simulink model "quadplane_control_dev"  (R2023a)
settings: Solver=FixedStepAuto  StartTime=0.0  StopTime=10.0  FixedStep=0.01  RelTol=1e-3
undefined symbols (not defined in the file or in its folder): Aircraft, DiscIntNeverNeededParam, framePeriod_s, frameRate_hz, InitCond
libraries: simulink x8, eeGeneralControl x6, slpidlib x3, fuzblock x1
(part 1 of 3)
settings Model: Creator=lagerprocessor  LastModifiedBy=redro
settings SolverCC: ZeroCrossControl=DisableAll
settings DataIOCC: SaveOutput=off  DSMLogging=off  SaveTime=off
settings DebuggingCC: ParameterPrecisionLossMsg=none
settings ModelReferenceCC: UseModelRefSolver=on
settings GRTTargetCC: CombineOutputUpdateFcns=off  MatFileLogging=off

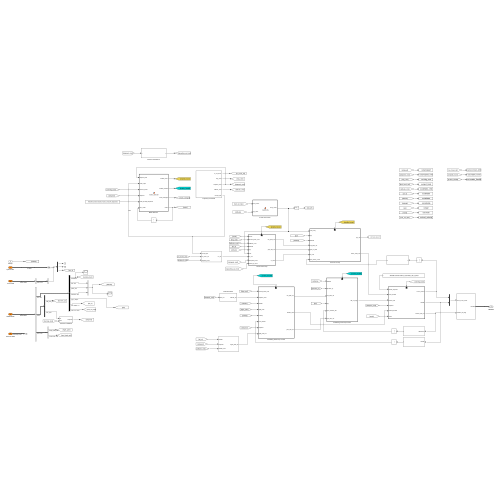
[thumbnail: Simulink's stored preview of the top-level diagram]
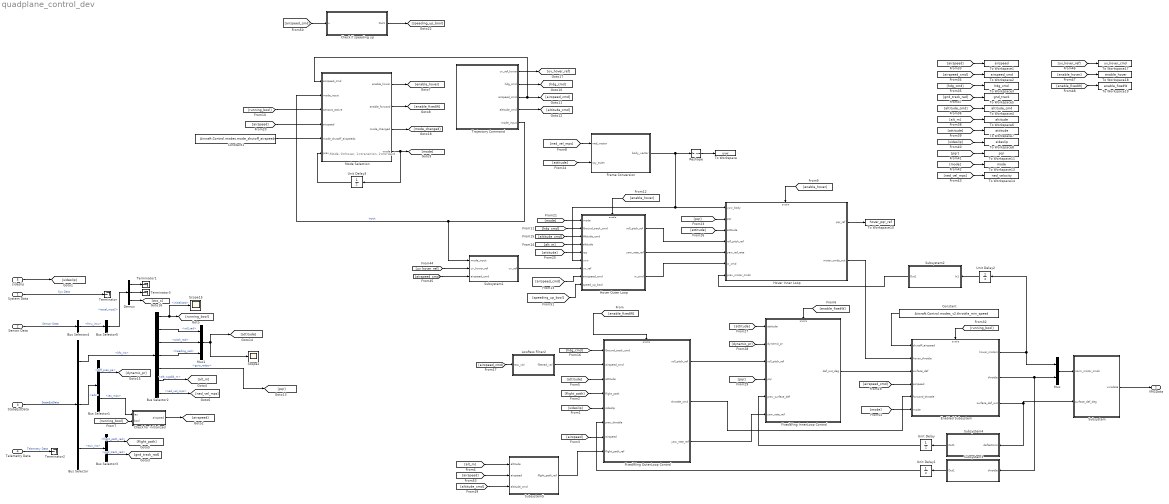
== system quadplane_control_dev ==
  note: Mode: 0=hover, 1=transition, 2=forward
  System Data : Inport  OutDataTypeStr=Bus: SysData  SampleTime=framePeriod_s  BusOutputAsStruct=on
  Sensor Data : Inport  Port=2  OutDataTypeStr=Bus: SensorData  SampleTime=framePeriod_s  BusOutputAsStruct=on
  StateEstData : Inport  Port=3  OutDataTypeStr=Bus: StateEstData  BusOutputAsStruct=on
  Telemetry Data : Inport  Port=4  OutDataTypeStr=Bus: TelemData  SampleTime=framePeriod_s  BusOutputAsStruct=on
  sideslip : Inport  Port=5  OutDataTypeStr=single
  Bus Selector : BusSelector  OutputSignals=bfs_ins,adc,aux_ins
  Bus Selector1 : BusSelector  OutputSignals=diff_pres_pa,ias_mps
  Bus Selector2 : BusSelector  OutputSignals=initialized,roll_rad,pitch_rad,heading_rad,gyro_radps,alt_wgs84_m,ned_vel_mps
  Bus Selector3 : BusSelector  OutputSignals=flight_path_rad,gnd_track_rad
  Bus Selector4 : BusSelector  OutputSignals=fmu_imu
  Bus Selector5 : BusSelector  OutputSignals=accel_mps2
  Check for initialized : Subsystem
  Check if speeding up : Subsystem
  Constant : Constant  Value=Aircraft.Control.modes_v2.throttle_min_speed
  Constant1 : Constant  Value=Aircraft.Control.modes.mode_shutoff_airspeeds
  Demux : Demux  Outputs=3
  Enabled Subsystem : Subsystem  TreatAsAtomicUnit=on
  FixedWing InnerLoop Control : Subsystem  TreatAsAtomicUnit=on
  FixedWing OuterLoop Control : Subsystem  TreatAsAtomicUnit=on
  Frame Conversion : MATLAB Function  TreatAsAtomicUnit=on
  Hover Inner Loop : Subsystem  TreatAsAtomicUnit=on
  Hover Outer Loop : Subsystem  TreatAsAtomicUnit=on
  LowPass Filter2 : Subsystem
      settings: PortSchema="{\"entries\":[{\"content\":{\"sides\":[{\"content\":{\"connectorIds\":[\"Out1\"]},\"type\":\"ConnectorPlacement.EquallySpacedRectSide\",\"uuid\":\"91cc3e13-2b14-472d-8884-d1975898cd34\"},{\"content\":{\"connectorIds\":[\"In1\"],\"side\":\"RIGHT\"},\"type\":\"ConnectorPlacement.EquallySpacedRectSide\",\"uuid\":\"ce6b3021-6e32-4737-8c8e-25014706d3dd\"},{\"content\":{\"side\":\"TOP\"},\"type\":\"ConnectorPlacement.EquallySpacedRectSide\",\"uuid\":\"ad734f0b-b067-43e6-a641-0e0955250a7f\"},{\"content\":{\"side\":\"BOTTOM\"},\"type\":\"ConnectorPlacement.EquallySpacedRectSide\",\"uuid\":\"618c62c8-d4e2-4678-9fe1-905e2f147d5d\"}]},\"type\":\"ConnectorPlacement.EquallySpacedConnector\",\"uuid\":\"c0097053-d36a-473a-84fb-0616f69f4bc5\"}],\"packageUris\":[\"http://schema.mathworks.com/mf0/Connector/R2020b\"],\"version\":\"1.0\"}"
  Mode Selection : MATLAB Function  TreatAsAtomicUnit=on
  Mux : Mux  Inputs=2
  Mux1 : Mux  Inputs=3
  Reshape : Reshape
  Scope15 : Scope
  Scope2 : Scope
  Subsystem : Subsystem
  Subsystem1 : Subsystem
  Subsystem2 : Subsystem
  Subsystem3 : Subsystem
  Subsystem4 : Subsystem
  Subsystem5 : Subsystem
  Terminator{,1..3} (4 alike) : Terminator
  To Workspace : ToWorkspace  VariableName=uvw  SampleTime=-1
      settings: Save2DSignal=2-D array (concatenate along first dimension)
  To Workspace1 : ToWorkspace  VariableName=airspeed  SaveFormat=Timeseries  SampleTime=-1
  To Workspace10 : ToWorkspace  VariableName=hover_pqr_ref  SaveFormat=Timeseries  SampleTime=-1
  To Workspace11 : ToWorkspace  VariableName=pqr  SaveFormat=Timeseries  SampleTime=-1
  To Workspace13 : ToWorkspace  VariableName=mode  SaveFormat=Timeseries  SampleTime=-1
  To Workspace14 : ToWorkspace  VariableName=ned_velocity  SaveFormat=Timeseries  SampleTime=-1
  To Workspace17 : ToWorkspace  VariableName=uv_hover_cmd  SaveFormat=Timeseries  SampleTime=-1
  To Workspace18 : ToWorkspace  VariableName=enable_hover  SaveFormat=Timeseries  SampleTime=-1
  To Workspace19 : ToWorkspace  VariableName=enable_fixedW  SaveFormat=Timeseries  SampleTime=-1
  To Workspace2 : ToWorkspace  VariableName=airspeed_cmd  SaveFormat=Timeseries  SampleTime=-1
  To Workspace3 : ToWorkspace  VariableName=hdg_cmd  SaveFormat=Timeseries  SampleTime=-1
  To Workspace4 : ToWorkspace  VariableName=altitude_cmd  SaveFormat=Timeseries  SampleTime=-1
  To Workspace5 : ToWorkspace  VariableName=gnd_track  SaveFormat=Timeseries  SampleTime=-1
  To Workspace6 : ToWorkspace  VariableName=altitude  SaveFormat=Timeseries  SampleTime=-1
  To Workspace7 : ToWorkspace  VariableName=attitude  SaveFormat=Timeseries  SampleTime=-1
  To Workspace8 : ToWorkspace  VariableName=sideslip  SaveFormat=Timeseries  SampleTime=-1
  Trajectory Command : Subsystem
  Unit Delay{,1..3} (4 alike) : UnitDelay  SampleTime=-1  HasFrameUpgradeWarning=on
  VMSData : Outport  OutDataTypeStr=Bus: VmsData
  wires:
  Telemetry Data/1 -> Terminator2/1  "Telemetry Data"
  StateEstData/1 -> Bus Selector/1  "StateEstData"
  Sensor Data/1 -> Bus Selector4/1  "Sensor Data"
  System Data/1 -> Terminator/1  "Sys Data"
  Subsystem/1(vmsdata) -> VMSData/1
  Bus Selector/2 -> Bus Selector1/1  "<adc>"
  Bus Selector/1 -> Bus Selector2/1  "<bfs_ins>"
  [enable_fixedW] -> FixedWing InnerLoop Control/Enable
  Bus Selector2/3 -> Mux1/2  "<pitch_rad>"
  Bus Selector2/4 -> Mux1/3  "<heading_rad>"
  Bus Selector/3 -> Bus Selector3/1  "<aux_ins>"
  Bus Selector4/1 -> Bus Selector5/1  "<fmu_imu>"
  Bus Selector5/1 -> Demux/1  "<accel_mps2>"
  Demux/1 -> Terminator1/1
  Demux/2 -> Terminator3/1
  sideslip/1 -> [sideslip]
  [sideslip] -> FixedWing OuterLoop Control/5(sideslip)
  Bus Selector2/1 -> Scope15/1, [running_bool]  "<initialized>"
  Bus Selector2/2 -> Mux1/1  "<roll_rad>"
  [hdg_cmd] -> FixedWing OuterLoop Control/1(Ground_track_cmd)
  Bus Selector3/2 -> [gnd_track_rad]  "<gnd_track_rad>"
  Bus Selector2/6 -> [alt_m]  "<alt_wgs84_m>"
  FixedWing OuterLoop Control/1(roll_pitch_ref) -> FixedWing InnerLoop Control/3(roll_pitch_ref)
  [airspeed_cmd] -> LowPass Filter2/1(raw_val)
  [flight_path] -> FixedWing OuterLoop Control/4(flight_path)
  [airspeed] -> FixedWing OuterLoop Control/7(airspeed)
  [attitude] -> FixedWing OuterLoop Control/3(attitude)
  [enable_fixedW] -> FixedWing OuterLoop Control/Enable
  Bus Selector2/7 -> [ned_vel_mps]  "<ned_vel_mps>"
  [ned_vel_mps] -> Frame Conversion/1(ned_vector)
  FixedWing InnerLoop Control/1(def_out_deg) -> Enabled Subsystem/3(surface_def)
  [enable_hover] -> Hover Inner Loop/Enable
  Hover Inner Loop/2(motor_cmds_out) -> Enabled Subsystem/2(hover_throttle)
  Hover Outer Loop/1(roll_pitch_ref) -> Hover Inner Loop/4(roll_pitch_ref)
  Hover Outer Loop/2(yaw_rate_ref) -> Hover Inner Loop/5(yaw_ref_rate)
  [enable_hover] -> Hover Outer Loop/Enable
  Hover Outer Loop/3(w_cmd) -> Hover Inner Loop/6(w_cmd)
  [hdg_cmd] -> Hover Outer Loop/2(Ground_track_cmd)
  [altitude_cmd] -> Hover Outer Loop/3(Altitude_cmd)
  [alt_m] -> Hover Outer Loop/4(altitude)
  Mode Selection/1(enable_hover) -> [enable_hover]
  Mode Selection/2(enable_forward) -> [enable_fixedW]
  [running_bool] -> Mode Selection/3(sensors_active)
  Trajectory Command/2(hdg_cmd) -> [hdg_cmd]
  Trajectory Command/4(altitude_cmd) -> [altitude_cmd]
  Trajectory Command/3(airspeed_cmd) -> Mode Selection/1(airspeed_cmd), [airspeed_cmd]
  [airspeed_cmd] -> Enabled Subsystem/4(airspeed)
  Mux/1 -> Subsystem/1(norm_motor_cmds)
  Enabled Subsystem/2(throttle) -> Subsystem3/1(throttle), Mux/2
  Unit Delay/1 -> FixedWing InnerLoop Control/5(prev_surface_def)
  Subsystem2/1(Out1) -> Hover Inner Loop/7(prev_motor_cmds)
  [airspeed] -> Mode Selection/4(airspeed)
  [mode] -> Hover Outer Loop/1(mode)
  Mode Selection/4(mode) -> Unit Delay3/1, [mode]
  Bus Selector2/5 -> [pqr]  "<gyro_radps>"
  Mux1/1 -> Scope2/1, [attitude]
  Bus Selector1/1 -> [dynamic_pr]  "<diff_pres_pa>"
  Bus Selector3/1 -> [flight_path]  "<flight_path_rad>"
  Demux/3 -> [acc_z]
  [attitude] -> Frame Conversion/2(rpy_euler)
  [attitude] -> Hover Outer Loop/5(rpy)
  [pqr] -> Hover Inner Loop/2(pqr)
  [attitude] -> Hover Inner Loop/3(attitude)
  [attitude] -> FixedWing InnerLoop Control/1(attitude)
  [dynamic_pr] -> FixedWing InnerLoop Control/2(dynamic_pr)
  [pqr] -> FixedWing InnerLoop Control/4(pqr)
  Bus Selector1/2 -> Check for initialized/1(ias)  "<ias_mps>"
  [running_bool] -> Enabled Subsystem/Enable
  Frame Conversion/1(body_vector) -> Reshape/1, Hover Inner Loop/1(uvw_body), Hover Outer Loop/6(uvw)
  [airspeed] -> To Workspace1/1
  [airspeed_cmd] -> To Workspace2/1
  [hdg_cmd] -> To Workspace3/1
  [altitude_cmd] -> To Workspace4/1
  [gnd_track_rad] -> To Workspace5/1
  [alt_m] -> To Workspace6/1
  [attitude] -> To Workspace7/1
  [sideslip] -> To Workspace8/1
  Hover Inner Loop/1(pqr_ref) -> To Workspace10/1
  [pqr] -> To Workspace11/1
  [mode] -> To Workspace13/1
  [ned_vel_mps] -> To Workspace14/1
  Trajectory Command/1(uv_ref_hover) -> [uv_hover_ref]
  Reshape/1 -> To Workspace/1
  Enabled Subsystem/1(hover_motors) -> Unit Delay2/1, Mux/1
  Enabled Subsystem/3(surface_def_out) -> Subsystem/2(surface_def_deg), Subsystem4/1(deflections)
  Subsystem1/1(uv_ref) -> Hover Outer Loop/7(uv_ref)
  [airspeed_cmd] -> Subsystem1/3(airspeed_cmd)
  [uv_hover_ref] -> Subsystem1/2(uv_hover_ref)
  [enable_hover] -> To Workspace18/1
  [enable_fixedW] -> To Workspace19/1
  [uv_hover_ref] -> To Workspace17/1
  FixedWing OuterLoop Control/3(yaw_rate_ref) -> FixedWing InnerLoop Control/6(yaw_rate_ref)
  Unit Delay2/1 -> Subsystem2/1(In1)
  Subsystem4/1(Out1) -> Unit Delay/1
  Unit Delay1/1 -> FixedWing OuterLoop Control/6(prev_throttle)
  Subsystem3/1(Out1) -> Unit Delay1/1
  Check for initialized/1(airspeed) -> [airspeed]
  [running_bool] -> Check for initialized/2(bool)
  Unit Delay3/1 -> Mode Selection/6(prev_mode)
  [mode] -> Enabled Subsystem/6(mode)
  Trajectory Command/5(mode_input) -> Subsystem1/1(mode_input), Mode Selection/2(mode_input)  "input"
  Mode Selection/3(mode_changed) -> [mode_changed]
  LowPass Filter2/1(filtered_val) -> FixedWing OuterLoop Control/2(airspeed_cmd)
  Constant/1 -> Enabled Subsystem/1(shutoff_airspeed)
  Constant1/1 -> Mode Selection/5(mode_shutoff_airspeeds)
  FixedWing OuterLoop Control/2(throttle_cmd) -> Enabled Subsystem/5(forward_throttle)
  [airspeed_cmd] -> Hover Outer Loop/8(airscpeed_cmd)
  [airspeed_cmd] -> Check if speeding up/1(u)
  Check if speeding up/1(Out1) -> [speeding_up_bool]
  [speeding_up_bool] -> Hover Outer Loop/9(speed_up_bool)
  [alt_m] -> Subsystem5/1(altitude)
  [altitude_cmd] -> Subsystem5/3(altitude_cmd)
  [airspeed] -> Subsystem5/2(airspeed)
  Subsystem5/1(flight_path_ref) -> FixedWing OuterLoop Control/8(flight_path_ref)

== system quadplane_control_dev/Check for initialized ==
  ias : Inport
  bool : Inport  Port=2
  Constant : Constant  Value=InitCond.body_vel_mps(1)  OutDataTypeStr=single
  Switch : Switch  Criteria=u2 > Threshold  SaturateOnIntegerOverflow=off  InputSameDT=off
  airspeed : Outport
  wires:
  ias/1 -> Switch/1
  bool/1 -> Switch/2  "bool"
  Constant/1 -> Switch/3
  Switch/1 -> airspeed/1

== system quadplane_control_dev/Check if speeding up ==
  u : Inport
  Constant2 : Constant  OutDataTypeStr=single
  Constant3 : Constant  Value=0  OutDataTypeStr=single
  Filtered Derivative (Discrete or Continuous) : eeGeneralControl/Filtered Derivative (Discrete or Continuous)  K=1  T=0.1  B=inf  A=-inf  minRatio=10  init_option=Inherited from block input  x0=0  Ts=-1
      settings: LibrarySourceBlock=|
      | ee_sl_lib/General Control/Filtered Derivative
      | (Discrete or Continuous)
  LowPass Filter : Subsystem
  Scope : Scope
  Switch : Switch  Criteria=u2 > Threshold  SaturateOnIntegerOverflow=off  InputSameDT=off
  Out1 : Outport
  wires:
  Filtered Derivative (Discrete or Continuous)/1 -> LowPass Filter/1(raw_val)
  Switch/1 -> Out1/1
  LowPass Filter/1(filtered_val) -> Scope/1, Switch/2
  Constant3/1 -> Switch/3
  Constant2/1 -> Switch/1
  u/1 -> Filtered Derivative (Discrete or Continuous)/1

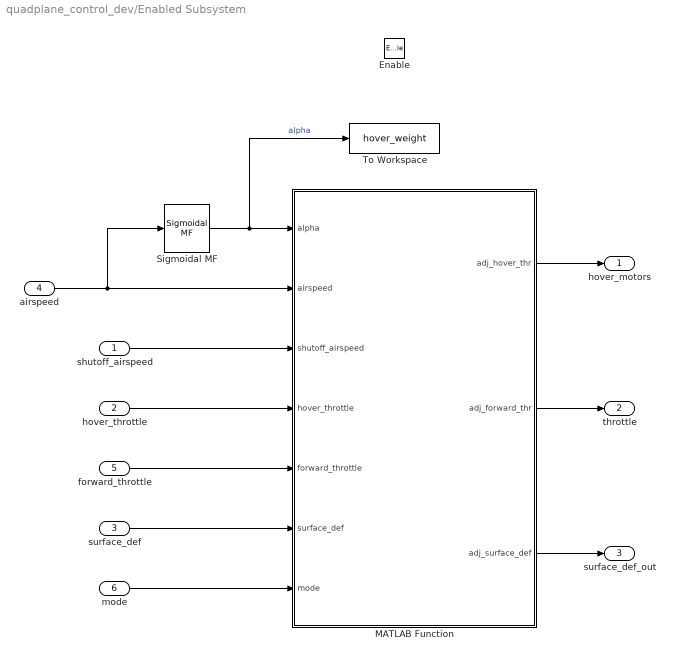
== system quadplane_control_dev/Enabled Subsystem ==
  shutoff_airspeed : Inport
  hover_throttle : Inport  Port=2
  surface_def : Inport  Port=3
  airspeed : Inport  Port=4
  forward_throttle : Inport  Port=5
  mode : Inport  Port=6
  Enable : EnablePort
  MATLAB Function : MATLAB Function  TreatAsAtomicUnit=on
  Sigmoidal MF : fuzblock/Membership  Functions/Sigmoidal MF  a=Aircraft.Control.modes_v2.transition_sigmoidal_a  c=Aircraft.Control.modes_v2.transition_sigmoidal_c
  To Workspace : ToWorkspace  VariableName=hover_weight  SaveFormat=Timeseries  SampleTime=-1
  hover_motors : Outport
  throttle : Outport  Port=2
  surface_def_out : Outport  Port=3
  wires:
  MATLAB Function/3(adj_surface_def) -> surface_def_out/1
  MATLAB Function/2(adj_forward_thr) -> throttle/1
  airspeed/1 -> Sigmoidal MF/1, MATLAB Function/2(airspeed)
  forward_throttle/1 -> MATLAB Function/5(forward_throttle)
  surface_def/1 -> MATLAB Function/6(surface_def)
  Sigmoidal MF/1 -> To Workspace/1, MATLAB Function/1(alpha)  "alpha"
  MATLAB Function/1(adj_hover_thr) -> hover_motors/1
  hover_throttle/1 -> MATLAB Function/4(hover_throttle)
  mode/1 -> MATLAB Function/7(mode)
  shutoff_airspeed/1 -> MATLAB Function/3(shutoff_airspeed)

== system quadplane_control_dev/FixedWing InnerLoop Control ==
  attitude : Inport
  dynamic_pr : Inport  Port=2
  roll_pitch_ref : Inport  Port=3
  pqr : Inport  Port=4
  prev_surface_def : Inport  Port=5
  yaw_rate_ref : Inport  Port=6
  Enable : EnablePort
  INDI Based Angular Rate Controller : Subsystem
  NDI based Attitude Controller : Subsystem
  To Workspace : ToWorkspace  VariableName=forward_pqr_cmd  SaveFormat=Timeseries  SampleTime=-1
  def_out_deg : Outport
  wires:
  dynamic_pr/1 -> INDI Based Angular Rate Controller/1(dynamic_pr)
  pqr/1 -> INDI Based Angular Rate Controller/3(pqr)
  attitude/1 -> NDI based Attitude Controller/1(attitude)
  NDI based Attitude Controller/1(pqr_ref) -> To Workspace/1, INDI Based Angular Rate Controller/2(pqr_ref)
  roll_pitch_ref/1 -> NDI based Attitude Controller/2(roll_pitch_ref)
  prev_surface_def/1 -> INDI Based Angular Rate Controller/4(prev_surface_def)
  INDI Based Angular Rate Controller/1(def_out_deg) -> def_out_deg/1
  yaw_rate_ref/1 -> NDI based Attitude Controller/3(yaw_rate_ref)

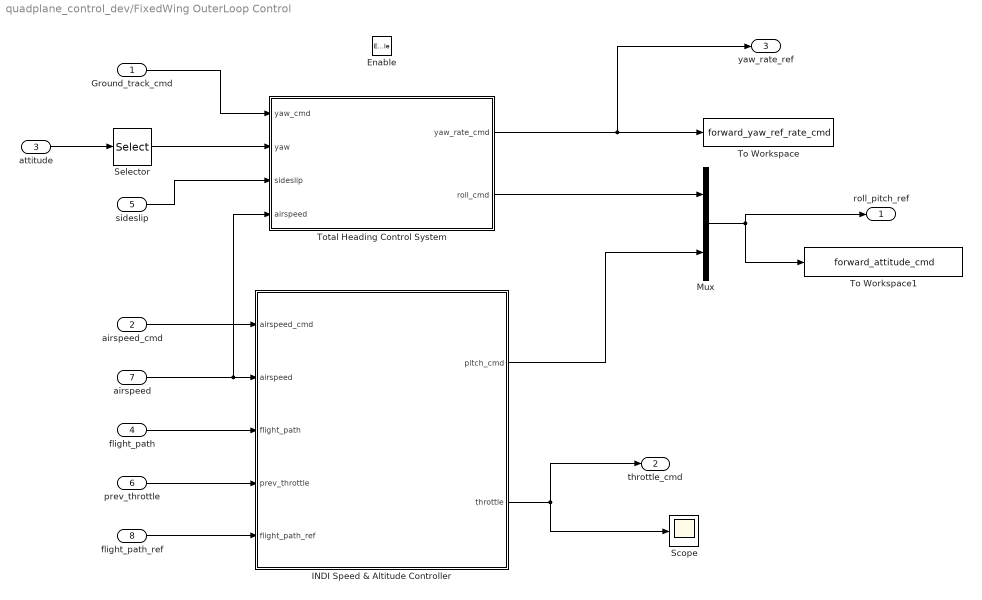
== system quadplane_control_dev/FixedWing OuterLoop Control ==
  Ground_track_cmd : Inport
  airspeed_cmd : Inport  Port=2
  attitude : Inport  Port=3
  flight_path : Inport  Port=4
  sideslip : Inport  Port=5
  prev_throttle : Inport  Port=6
  airspeed : Inport  Port=7
  flight_path_ref : Inport  Port=8
  Enable : EnablePort
  INDI Speed & Altitude Controller : Subsystem
  Mux : Mux  Inputs=2
  Scope : Scope
  Selector : Selector  InputPortWidth=3  IndexOptions=Index vector (dialog)  Indices=3  OutputSizes=1
  To Workspace : ToWorkspace  VariableName=forward_yaw_ref_rate_cmd  SaveFormat=Timeseries  SampleTime=-1
  To Workspace1 : ToWorkspace  VariableName=forward_attitude_cmd  SaveFormat=Timeseries  SampleTime=-1
  Total Heading Control System : Subsystem
  roll_pitch_ref : Outport
  throttle_cmd : Outport  Port=2
  yaw_rate_ref : Outport  Port=3
  wires:
  Ground_track_cmd/1 -> Total Heading Control System/1(yaw_cmd)
  INDI Speed & Altitude Controller/2(throttle) -> throttle_cmd/1, Scope/1
  flight_path/1 -> INDI Speed & Altitude Controller/3(flight_path)
  airspeed/1 -> Total Heading Control System/4(airspeed), INDI Speed & Altitude Controller/2(airspeed)
  Selector/1 -> Total Heading Control System/2(yaw)
  attitude/1 -> Selector/1
  sideslip/1 -> Total Heading Control System/3(sideslip)
  Mux/1 -> roll_pitch_ref/1, To Workspace1/1
  Total Heading Control System/2(roll_cmd) -> Mux/1
  Total Heading Control System/1(yaw_rate_cmd) -> yaw_rate_ref/1, To Workspace/1
  prev_throttle/1 -> INDI Speed & Altitude Controller/4(prev_throttle)
  airspeed_cmd/1 -> INDI Speed & Altitude Controller/1(airspeed_cmd)
  INDI Speed & Altitude Controller/1(pitch_cmd) -> Mux/2
  flight_path_ref/1 -> INDI Speed & Altitude Controller/5(flight_path_ref)

== system quadplane_control_dev/Hover Inner Loop ==
  uvw_body : Inport
  pqr : Inport  Port=2
  attitude : Inport  Port=3
  roll_pitch_ref : Inport  Port=4
  yaw_ref_rate : Inport  Port=5
  w_cmd : Inport  Port=6
  prev_motor_cmds : Inport  Port=7
  Enable : EnablePort
  Attitude Control : Subsystem
  INDI inner loop : Subsystem
  pqr_ref : Outport
  motor_cmds_out : Outport  Port=2
  wires:
  Attitude Control/1(pqr_ref1) -> pqr_ref/1, INDI inner loop/1(pqr_ref)
  uvw_body/1 -> INDI inner loop/2(uvw_body)
  pqr/1 -> INDI inner loop/4(pqr)
  INDI inner loop/1(motor_cmds_out) -> motor_cmds_out/1
  attitude/1 -> Attitude Control/3(roll_pitch_yaw)
  roll_pitch_ref/1 -> Attitude Control/2(roll_pitch_ref)
  prev_motor_cmds/1 -> INDI inner loop/5(prev_motor_cmds)
  w_cmd/1 -> INDI inner loop/3(w_ref)
  yaw_ref_rate/1 -> Attitude Control/1(yaw_rate_ref)

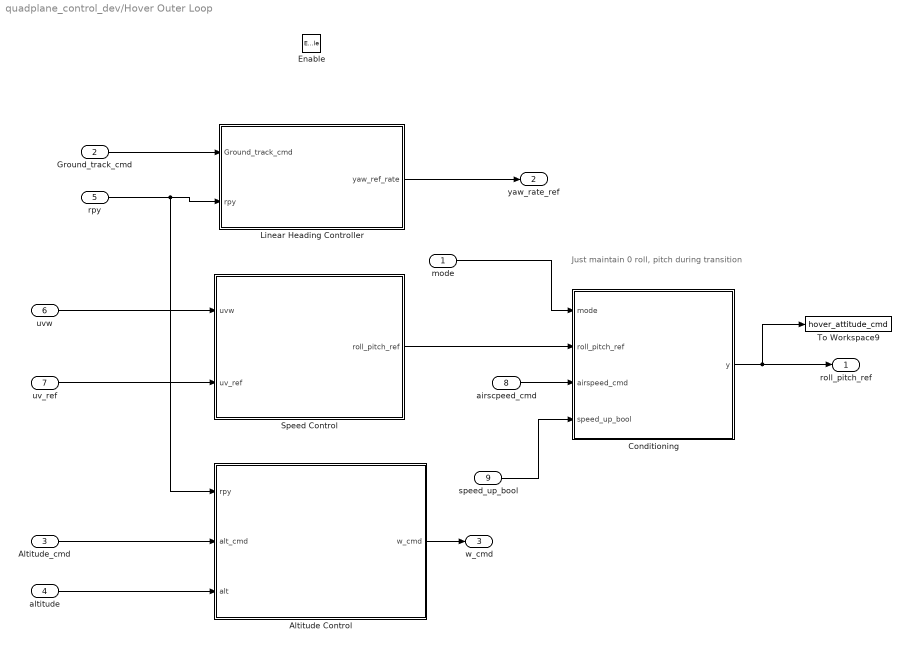
== system quadplane_control_dev/Hover Outer Loop ==
  note: Just maintain 0 roll, pitch during transition
  mode : Inport
  Ground_track_cmd : Inport  Port=2
  Altitude_cmd : Inport  Port=3
  altitude : Inport  Port=4
  rpy : Inport  Port=5
  uvw : Inport  Port=6
  uv_ref : Inport  Port=7
  airscpeed_cmd : Inport  Port=8
  speed_up_bool : Inport  Port=9
  Enable : EnablePort
  Altitude Control : Subsystem
  Conditioning : Subsystem
  Linear Heading Controller : Subsystem
  Speed Control : Subsystem
  To Workspace9 : ToWorkspace  VariableName=hover_attitude_cmd  SaveFormat=Timeseries  SampleTime=-1
  roll_pitch_ref : Outport
  yaw_rate_ref : Outport  Port=2
  w_cmd : Outport  Port=3
  wires:
  Altitude_cmd/1 -> Altitude Control/2(alt_cmd)
  altitude/1 -> Altitude Control/3(alt)
  rpy/1 -> Linear Heading Controller/2(rpy), Altitude Control/1(rpy)
  uvw/1 -> Speed Control/1(uvw)
  Speed Control/1(roll_pitch_ref) -> Conditioning/2(roll_pitch_ref)
  Altitude Control/1(w_cmd) -> w_cmd/1
  Conditioning/1(y) -> To Workspace9/1, roll_pitch_ref/1
  uv_ref/1 -> Speed Control/2(uv_ref)
  Linear Heading Controller/1(yaw_ref_rate) -> yaw_rate_ref/1
  Ground_track_cmd/1 -> Linear Heading Controller/1(Ground_track_cmd)
  mode/1 -> Conditioning/1(mode)
  airscpeed_cmd/1 -> Conditioning/3(airspeed_cmd)
  speed_up_bool/1 -> Conditioning/4(speed_up_bool)

== system quadplane_control_dev/LowPass Filter2 ==
  raw_val : Inport
  Constant : Constant  Value=Aircraft.Control.Forward_v2.airspeed_ref_LP_filter_CTOFF
  LP Filter on throttle outputs : Subsystem
      settings: PortSchema="{\"entries\":[{\"content\":{\"sides\":[{\"content\":{\"connectorIds\":[\"In1\"]},\"type\":\"ConnectorPlacement.EquallySpacedRectSide\",\"uuid\":\"20236834-aeb3-4c5b-bb2e-f84447e752b5\"},{\"content\":{\"connectorIds\":[\"Out1\"],\"side\":\"RIGHT\"},\"type\":\"ConnectorPlacement.EquallySpacedRectSide\",\"uuid\":\"d668f9a1-a3df-4207-8bf1-99fb838e59b2\"},{\"content\":{\"connectorIds\":[],\"side\":\"TOP\"},\"type\":\"ConnectorPlacement.EquallySpacedRectSide\",\"uuid\":\"66cceb06-f4bc-4278-b965-2427292e46df\"},{\"content\":{\"connectorIds\":[\"In2\"],\"side\":\"BOTTOM\"},\"type\":\"ConnectorPlacement.EquallySpacedRectSide\",\"uuid\":\"8fdaac6a-cb03-4bd4-87bb-7bafd10bc297\"}]},\"type\":\"ConnectorPlacement.EquallySpacedConnector\",\"uuid\":\"3dc29a9a-e794-478d-b7df-452e6c2d3f66\"}],\"packageUris\":[\"http://schema.mathworks.com/mf0/Connector/R2020b\"],\"version\":\"1.0\"}"
  To Workspace : ToWorkspace  VariableName=airspeed_ref  SaveFormat=Timeseries  SampleTime=-1
  filtered_val : Outport
  wires:
  raw_val/1 -> LP Filter on throttle outputs/1(raw_val)
  Constant/1 -> LP Filter on throttle outputs/2(freq_cut)
  LP Filter on throttle outputs/1(filtered_val) -> To Workspace/1, filtered_val/1

== system quadplane_control_dev/Subsystem ==
  note: norm_motor_cmds = [0,1]
  note: surface_def = [-30, 30]
  norm_motor_cmds : Inport
  surface_def_deg : Inport  Port=2
  Subsystem1 : Subsystem
  deflections_PWM_denormalize : Subsystem
  motor_PWM_denormalize : Subsystem
  vmsdata : Outport
  wires:
  motor_PWM_denormalize/1(raw_output) -> Subsystem1/1(Motor_Cmds)
  deflections_PWM_denormalize/1(raw_output) -> Subsystem1/2(Surface_def)
  Subsystem1/1(vmsdata) -> vmsdata/1
  norm_motor_cmds/1 -> motor_PWM_denormalize/1(normalized_input)
  surface_def_deg/1 -> deflections_PWM_denormalize/1(normalized_input)

== system quadplane_control_dev/Subsystem1 ==
  mode_input : Inport
  uv_hover_ref : Inport  Port=2
  airspeed_cmd : Inport  Port=3
  Constant : Constant  Value=0  OutDataTypeStr=single
  LowPass Filter1 : Subsystem
      settings: PortSchema="{\"entries\":[{\"content\":{\"sides\":[{\"content\":{\"connectorIds\":[\"Out1\"]},\"type\":\"ConnectorPlacement.EquallySpacedRectSide\",\"uuid\":\"91cc3e13-2b14-472d-8884-d1975898cd34\"},{\"content\":{\"connectorIds\":[\"In1\"],\"side\":\"RIGHT\"},\"type\":\"ConnectorPlacement.EquallySpacedRectSide\",\"uuid\":\"ce6b3021-6e32-4737-8c8e-25014706d3dd\"},{\"content\":{\"side\":\"TOP\"},\"type\":\"ConnectorPlacement.EquallySpacedRectSide\",\"uuid\":\"ad734f0b-b067-43e6-a641-0e0955250a7f\"},{\"content\":{\"side\":\"BOTTOM\"},\"type\":\"ConnectorPlacement.EquallySpacedRectSide\",\"uuid\":\"618c62c8-d4e2-4678-9fe1-905e2f147d5d\"}]},\"type\":\"ConnectorPlacement.EquallySpacedConnector\",\"uuid\":\"c0097053-d36a-473a-84fb-0616f69f4bc5\"}],\"packageUris\":[\"http://schema.mathworks.com/mf0/Connector/R2020b\"],\"version\":\"1.0\"}"
  Mux : Mux  Inputs=2
  Switch : Switch  Criteria=u2 > Threshold  SaturateOnIntegerOverflow=off  InputSameDT=off
  To Workspace : ToWorkspace  VariableName=uv_ref  SaveFormat=Timeseries  SampleTime=-1
  uv_ref : Outport
  wires:
  Switch/1 -> LowPass Filter1/1(raw_val)
  mode_input/1 -> Switch/2
  airspeed_cmd/1 -> Mux/1
  Constant/1 -> Mux/2
  Mux/1 -> Switch/1
  uv_hover_ref/1 -> Switch/3
  LowPass Filter1/1(filtered_val) -> To Workspace/1, uv_ref/1

== system quadplane_control_dev/Subsystem2 ==
  In1 : Inport
  Cast To Double : DataTypeConversion  OutDataTypeStr=double  SaturateOnIntegerOverflow=off  RndMeth=Floor
  Cast To Single : DataTypeConversion  OutDataTypeStr=single  SaturateOnIntegerOverflow=off  RndMeth=Floor
  Demux1 : Demux
  Mux2 : Mux
  Transfer Fcn{,1..3} (4 alike) : TransferFcn  Denominator=[1/Aircraft.Motor.bandwidth 1]
  Out1 : Outport
  wires:
  Transfer Fcn/1 -> Mux2/1
  Mux2/1 -> Cast To Single/1
  Transfer Fcn3/1 -> Mux2/4
  Demux1/2 -> Transfer Fcn1/1
  Demux1/3 -> Transfer Fcn2/1
  Demux1/4 -> Transfer Fcn3/1
  Transfer Fcn2/1 -> Mux2/3
  Transfer Fcn1/1 -> Mux2/2
  Demux1/1 -> Transfer Fcn/1
  In1/1 -> Cast To Double/1
  Cast To Double/1 -> Demux1/1
  Cast To Single/1 -> Out1/1

== system quadplane_control_dev/Subsystem3 ==
  throttle : Inport
  Cast To Double : DataTypeConversion  OutDataTypeStr=double  SaturateOnIntegerOverflow=off  RndMeth=Floor
  Cast To Single : DataTypeConversion  OutDataTypeStr=single  SaturateOnIntegerOverflow=off  RndMeth=Floor
  Transfer Fcn2 : TransferFcn  Denominator=[1/Aircraft.Motor.bandwidth 1]
  Out1 : Outport
  wires:
  throttle/1 -> Cast To Double/1
  Cast To Single/1 -> Out1/1
  Transfer Fcn2/1 -> Cast To Single/1
  Cast To Double/1 -> Transfer Fcn2/1

== system quadplane_control_dev/Subsystem4 ==
  deflections : Inport
  Cast To Double : DataTypeConversion  OutDataTypeStr=double  SaturateOnIntegerOverflow=off  RndMeth=Floor
  Cast To Single : DataTypeConversion  OutDataTypeStr=single  SaturateOnIntegerOverflow=off  RndMeth=Floor
  Demux : Demux  Outputs=3
  Mux : Mux  Inputs=3
  Transfer Fcn : TransferFcn  Denominator=[Aircraft.Surf.time_constant 1]
  Transfer Fcn1 : TransferFcn  Denominator=[Aircraft.Surf.time_constant 1]
  Transfer Fcn2 : TransferFcn  Denominator=[Aircraft.Surf.time_constant 1]
  Out1 : Outport
  wires:
  deflections/1 -> Cast To Double/1
  Cast To Single/1 -> Out1/1
  Transfer Fcn2/1 -> Mux/3
  Mux/1 -> Cast To Single/1
  Demux/2 -> Transfer Fcn1/1
  Demux/1 -> Transfer Fcn/1
  Transfer Fcn/1 -> Mux/1
  Demux/3 -> Transfer Fcn2/1
  Transfer Fcn1/1 -> Mux/2
  Cast To Double/1 -> Demux/1

== system quadplane_control_dev/Subsystem5 ==
  note: Converting from Alt_cmd to Flight_path_cmd
  altitude : Inport
  airspeed : Inport  Port=2
  altitude_cmd : Inport  Port=3
  Asin : Trigonometry  Operator=asin
  Divide : Product  Inputs=/*
  Gain : Gain  Gain=Aircraft.Control.Forward_v2.altitude_P
  LowPass Filter1 : Subsystem
      settings: PortSchema="{\"entries\":[{\"content\":{\"sides\":[{\"content\":{\"connectorIds\":[\"Out1\"]},\"type\":\"ConnectorPlacement.EquallySpacedRectSide\",\"uuid\":\"91cc3e13-2b14-472d-8884-d1975898cd34\"},{\"content\":{\"connectorIds\":[\"In1\"],\"side\":\"RIGHT\"},\"type\":\"ConnectorPlacement.EquallySpacedRectSide\",\"uuid\":\"ce6b3021-6e32-4737-8c8e-25014706d3dd\"},{\"content\":{\"side\":\"TOP\"},\"type\":\"ConnectorPlacement.EquallySpacedRectSide\",\"uuid\":\"ad734f0b-b067-43e6-a641-0e0955250a7f\"},{\"content\":{\"side\":\"BOTTOM\"},\"type\":\"ConnectorPlacement.EquallySpacedRectSide\",\"uuid\":\"618c62c8-d4e2-4678-9fe1-905e2f147d5d\"}]},\"type\":\"ConnectorPlacement.EquallySpacedConnector\",\"uuid\":\"c0097053-d36a-473a-84fb-0616f69f4bc5\"}],\"packageUris\":[\"http://schema.mathworks.com/mf0/Connector/R2020b\"],\"version\":\"1.0\"}"
  Saturation1 : Saturate  UpperLimit=4  LowerLimit=-4
  Sum : Sum  Inputs=|+-
  To Workspace : ToWorkspace  VariableName=flight_path_ref  SaveFormat=Timeseries  SampleTime=-1
  flight_path_ref : Outport
  wires:
  Saturation1/1 -> Divide/2  "h_dot_cmd"
  Sum/1 -> Gain/1  "alt_err"
  Asin/1 -> LowPass Filter1/1(raw_val)  "flight_path_cmd"
  altitude_cmd/1 -> Sum/1
  airspeed/1 -> Divide/1
  Gain/1 -> Saturation1/1  "alt_err"
  Divide/1 -> Asin/1
  altitude/1 -> Sum/2
  LowPass Filter1/1(filtered_val) -> To Workspace/1, flight_path_ref/1

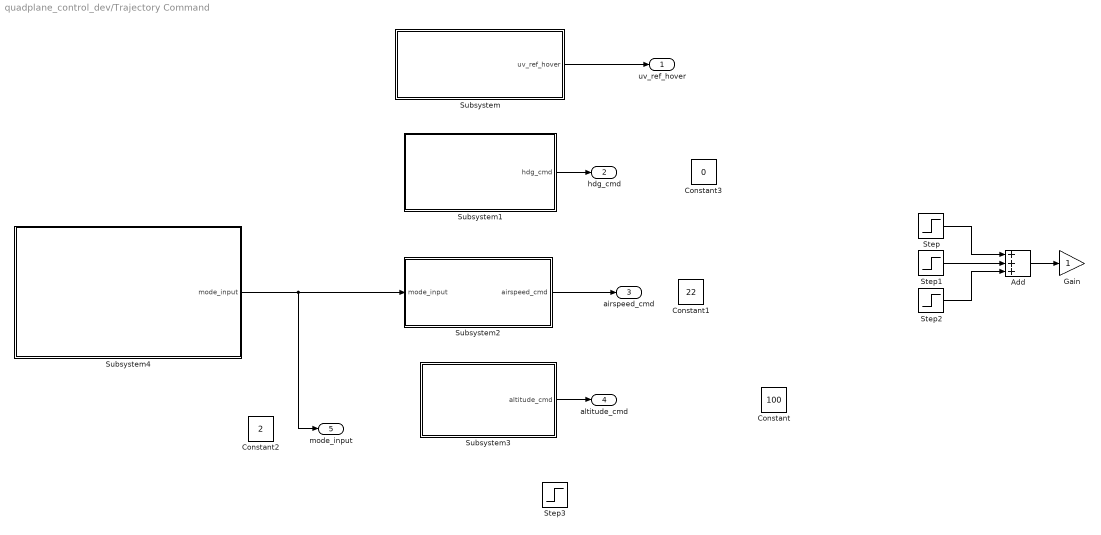
== system quadplane_control_dev/Trajectory Command ==
  Add : Sum  Inputs=+++
  Constant : Constant  Value=100  OutDataTypeStr=single
  Constant1 : Constant  Value=22  OutDataTypeStr=single
  Constant2 : Constant  Value=2  OutDataTypeStr=single
  Constant3 : Constant  Value=0  OutDataTypeStr=single
  Gain : Gain
  Step : Step  Time=6  OutDataTypeStr=single  SampleTime=0
  Step1 : Step  Time=12  Before=1  After=-1  OutDataTypeStr=single  SampleTime=0
  Step2 : Step  Time=18  Before=-1  After=0  OutDataTypeStr=single  SampleTime=0
  Step3 : Step  Time=3  Before=100  After=90  OutDataTypeStr=single  SampleTime=0
  Subsystem : Subsystem
  Subsystem1 : Subsystem
  Subsystem2 : Subsystem
  Subsystem3 : Subsystem
  Subsystem4 : Subsystem
  uv_ref_hover : Outport
  hdg_cmd : Outport  Port=2
  airspeed_cmd : Outport  Port=3
  altitude_cmd : Outport  Port=4
  mode_input : Outport  Port=5
  wires:
  Subsystem/1(uv_ref_hover) -> uv_ref_hover/1
  Subsystem3/1(altitude_cmd) -> altitude_cmd/1
  Subsystem4/1(mode_input) -> Subsystem2/1(mode_input), mode_input/1
  Subsystem2/1(airspeed_cmd) -> airspeed_cmd/1
  Subsystem1/1(hdg_cmd) -> hdg_cmd/1
  Step2/1 -> Add/3
  Step1/1 -> Add/2
  Step/1 -> Add/1
  Add/1 -> Gain/1

== system quadplane_control_dev/Check if speeding up/LowPass Filter ==
  raw_val : Inport
  Constant : Constant  Value=0.5  OutDataTypeStr=single
  LP Filter on Accel : Subsystem
      settings: PortSchema="{\"entries\":[{\"content\":{\"sides\":[{\"content\":{\"connectorIds\":[\"In1\"]},\"type\":\"ConnectorPlacement.EquallySpacedRectSide\",\"uuid\":\"20236834-aeb3-4c5b-bb2e-f84447e752b5\"},{\"content\":{\"connectorIds\":[\"Out1\"],\"side\":\"RIGHT\"},\"type\":\"ConnectorPlacement.EquallySpacedRectSide\",\"uuid\":\"d668f9a1-a3df-4207-8bf1-99fb838e59b2\"},{\"content\":{\"connectorIds\":[],\"side\":\"TOP\"},\"type\":\"ConnectorPlacement.EquallySpacedRectSide\",\"uuid\":\"66cceb06-f4bc-4278-b965-2427292e46df\"},{\"content\":{\"connectorIds\":[\"In2\"],\"side\":\"BOTTOM\"},\"type\":\"ConnectorPlacement.EquallySpacedRectSide\",\"uuid\":\"8fdaac6a-cb03-4bd4-87bb-7bafd10bc297\"}]},\"type\":\"ConnectorPlacement.EquallySpacedConnector\",\"uuid\":\"3dc29a9a-e794-478d-b7df-452e6c2d3f66\"}],\"packageUris\":[\"http://schema.mathworks.com/mf0/Connector/R2020b\"],\"version\":\"1.0\"}"
  filtered_val : Outport
  wires:
  raw_val/1 -> LP Filter on Accel/1(raw_val)
  Constant/1 -> LP Filter on Accel/2(freq_cut)
  LP Filter on Accel/1(filtered_val) -> filtered_val/1

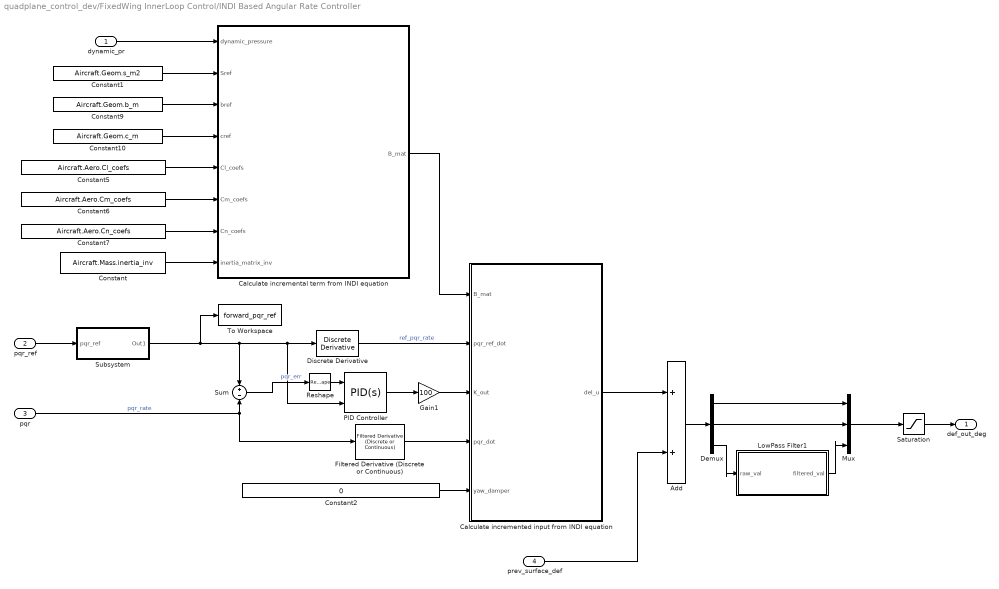
== system quadplane_control_dev/FixedWing InnerLoop Control/INDI Based Angular Rate Controller ==
  dynamic_pr : Inport
  pqr_ref : Inport  Port=2
  pqr : Inport  Port=3
  prev_surface_def : Inport  Port=4
  Add : Sum  OutDataTypeStr=single
  Calculate incremental term from INDI equation : MATLAB Function  TreatAsAtomicUnit=on
  Calculate incremented input from INDI equation : MATLAB Function  TreatAsAtomicUnit=on
  Constant : Constant  Value=Aircraft.Mass.inertia_inv  OutDataTypeStr=single
  Constant1 : Constant  Value=Aircraft.Geom.s_m2  OutDataTypeStr=single
  Constant10 : Constant  Value=Aircraft.Geom.c_m  OutDataTypeStr=single
  Constant2 : Constant  Value=0  OutDataTypeStr=single
  Constant5 : Constant  Value=Aircraft.Aero.Cl_coefs  OutDataTypeStr=single
  Constant6 : Constant  Value=Aircraft.Aero.Cm_coefs  OutDataTypeStr=single
  Constant7 : Constant  Value=Aircraft.Aero.Cn_coefs  OutDataTypeStr=single
  Constant9 : Constant  Value=Aircraft.Geom.b_m  OutDataTypeStr=single
  Demux : Demux  Outputs=3
  Discrete Derivative : simulink/Discrete/Discrete Derivative  gainval=1.0  ICPrevScaledInput=0.0  OutMin=[]  OutMax=[]  OutDataTypeStr=single  OutputDataTypeScalingMode=single  OutDataType=fixdt(1, 16)  OutScaling=2^-10  DoSatur=off
  Filtered Derivative (Discrete or Continuous) : eeGeneralControl/Filtered Derivative (Discrete or Continuous)  K=1  T=0.01  B=inf  A=-inf  minRatio=10  init_option=Inherited from block input  x0=0  Ts=-1
      settings: LibrarySourceBlock=|
      | ee_sl_lib/General Control/Filtered Derivative
      | (Discrete or Continuous)
  Gain1 : Gain  Gain=100
  LowPass Filter1 : Subsystem
      settings: PortSchema="{\"entries\":[{\"content\":{\"sides\":[{\"content\":{\"connectorIds\":[\"Out1\"]},\"type\":\"ConnectorPlacement.EquallySpacedRectSide\",\"uuid\":\"91cc3e13-2b14-472d-8884-d1975898cd34\"},{\"content\":{\"connectorIds\":[\"In1\"],\"side\":\"RIGHT\"},\"type\":\"ConnectorPlacement.EquallySpacedRectSide\",\"uuid\":\"ce6b3021-6e32-4737-8c8e-25014706d3dd\"},{\"content\":{\"side\":\"TOP\"},\"type\":\"ConnectorPlacement.EquallySpacedRectSide\",\"uuid\":\"ad734f0b-b067-43e6-a641-0e0955250a7f\"},{\"content\":{\"side\":\"BOTTOM\"},\"type\":\"ConnectorPlacement.EquallySpacedRectSide\",\"uuid\":\"618c62c8-d4e2-4678-9fe1-905e2f147d5d\"}]},\"type\":\"ConnectorPlacement.EquallySpacedConnector\",\"uuid\":\"c0097053-d36a-473a-84fb-0616f69f4bc5\"}],\"packageUris\":[\"http://schema.mathworks.com/mf0/Connector/R2020b\"],\"version\":\"1.0\"}"
  Mux : Mux  Inputs=3
  PID Controller : slpidlib/PID Controller  Controller=PID  Form=Parallel  TimeDomain=Continuous-time  UseExternalTs=off  SampleTime=-1  IntegratorMethod=Forward Euler  FilterMethod=Forward Euler  ControllerParametersSource=internal  P=[6, 6, 3]  I=[20, 20, 5]  UseKiTs=off  D=[0.5, 0.5, 0.75]  N=100  UseFilter=on  TunerSelectOption=Transfer Function Based (PID Tuner App)  InitialConditionSource=internal  InitialConditionForIntegrator=0  InitialConditionForFilter=0  DifferentiatorICPrevScaledInput=0  ExternalReset=none  TrackingMode=on  Kt=1  LimitOutput=off  SatLimitsSource=internal  UpperSaturationLimit=inf  LowerSaturationLimit=-inf  LinearizeAsGain=on  AntiWindupMode=none  Kb=1  LimitIntegrator=off  UpperIntegratorSaturationLimit=inf  LowerIntegratorSaturationLimit=-inf  POutMin=[]  POutMax=[]  IOutMin=[]  IOutMax=[]  DOutMin=[]  DOutMax=[]  NOutMin=[]  NOutMax=[]  SumOutMin=[]  SumOutMax=[]  SaturationOutMin=[]  SaturationOutMax=[]  PParamMin=[]  PParamMax=[]  IParamMin=[]  IParamMax=[]  DParamMin=[]  DParamMax=[]  NParamMin=[]  NParamMax=[]  KbParamMin=[]  KbParamMax=[]  KtParamMin=[]  KtParamMax=[]  KbOutMin=[]  KbOutMax=[]  KtOutMin=[]  KtOutMax=[]  IntegratorOutMin=[]  IntegratorOutMax=[]  FilterOutMin=[]  FilterOutMax=[]  SumI1OutMin=[]  SumI1OutMax=[]  SumI2OutMin=[]  SumI2OutMax=[]  SumI3OutMin=[]  SumI3OutMax=[]  SumI4OutMin=[]  SumI4OutMax=[]  SumDOutMin=[]  SumDOutMax=[]  DifferentiatorOutMin=[]  DifferentiatorOutMax=[]  FilterDiffOutCoefMin=[]  FilterDiffOutCoefMax=[]  ReciprocalOutMin=[]  ReciprocalOutMax=[]  SumDenOutMin=[]  SumDenOutMax=[]  SumNumOutMin=[]  SumNumOutMax=[]  DivideOutMin=[]  DivideOutMax=[]  UdiffTsProdOutMin=[]  UdiffTsProdOutMax=[]  NTsProdOutMin=[]  NTsProdOutMax=[]  UintegralTsProdOutMin=[]  UintegralTsProdOutMax=[]  UngainTsProdOutMin=[]  UngainTsProdOutMax=[]  ClampingZeroOutDataTypeStr=Inherit: Inherit via back propagation  ClampingZeroOutMin=[]  ClampingZeroOutMax=[]  FilterDenConstantOutDataTypeStr=Inherit: Inherit via back propagation  FilterDenConstantOutMin=[]  FilterDenConstantOutMax=[]  PCopyOutDataTypeStr=Inherit: Inherit via back propagation  PCopyOutMin=[]  PCopyOutMax=[]  NCopyOutDataTypeStr=Inherit: Inherit via back propagation  NCopyOutMin=[]  NCopyOutMax=[]  IntegratorContinuousStateAttributes=''  IntegratorStateMustResolveToSignalObject=off  IntegratorRTWStateStorageClass=Auto  FilterContinuousStateAttributes=''  FilterStateMustResolveToSignalObject=off  FilterRTWStateStorageClass=Auto  ParallelPVariant=InternalParameters  IdealPVariant=Disabled  IVariant=InternalParameters  DVariant=InternalParameters  IntegratorVariant=Continuous  SatVariant=Disabled  AWVariant=Passthrough  PCopyVariant=Disabled  TRVariant=Enabled  FdbkBlocksVariant=Forward  IdealPFdbkVariant=Disabled  SatFdbkVariant=Disabled  DerivativeFilterVariant=ContFilter  NVariant=InternalParameters  NCopyVariant=Disabled  FilterICVariant=InternalICsFilter  IntegratorICVariant=InternalICs  ExternalResetVariant=Disabled  TRSumVariant=TrackingMode  SumFdbkVariant=Disabled  SumVariant=Sum_PID  TsampFilterVariant=InternalTs  TsampNgainVariant=Passthrough  TsampIntegralVariant=Disabled_SignalSpec  ExternalSaturationOutDataTypeStr=Inherit: Same as second input
  Reshape : Reshape
  Saturation : Saturate  UpperLimit=Aircraft.Surf.Limit.pos_deg  LowerLimit=Aircraft.Surf.Limit.neg_deg  OutDataTypeStr=single
  Subsystem : Subsystem
  Sum : Sum  Inputs=+-
  To Workspace : ToWorkspace  VariableName=forward_pqr_ref  SaveFormat=Timeseries  SampleTime=-1
  def_out_deg : Outport
  wires:
  pqr/1 -> Filtered Derivative (Discrete or Continuous)/1, Sum/2  "pqr_rate"
  Constant2/1 -> Calculate incremented input from INDI equation/5(yaw_damper)
  Constant7/1 -> Calculate incremental term from INDI equation/7(Cn_coefs)
  Discrete Derivative/1 -> Calculate incremented input from INDI equation/2(pqr_ref_dot)  "ref_pqr_rate"
  Saturation/1 -> def_out_deg/1
  dynamic_pr/1 -> Calculate incremental term from INDI equation/1(dynamic_pressure)
  Constant1/1 -> Calculate incremental term from INDI equation/2(Sref)
  Constant10/1 -> Calculate incremental term from INDI equation/4(cref)
  Constant6/1 -> Calculate incremental term from INDI equation/6(Cm_coefs)
  Sum/1 -> Reshape/1  "pqr_err"
  Constant5/1 -> Calculate incremental term from INDI equation/5(Cl_coefs)
  Constant/1 -> Calculate incremental term from INDI equation/8(inertia_matrix_inv)
  Constant9/1 -> Calculate incremental term from INDI equation/3(bref)
  Calculate incremental term from INDI equation/1(B_mat) -> Calculate incremented input from INDI equation/1(B_mat)
  Subsystem/1(Out1) -> To Workspace/1, PID Controller/2, Discrete Derivative/1, Sum/1
  prev_surface_def/1 -> Add/2
  PID Controller/1 -> Gain1/1
  Calculate incremented input from INDI equation/1(del_u) -> Add/1
  Add/1 -> Demux/1
  Filtered Derivative (Discrete or Continuous)/1 -> Calculate incremented input from INDI equation/4(pqr_dot)
  Mux/1 -> Saturation/1
  Gain1/1 -> Calculate incremented input from INDI equation/3(K_out)
  Reshape/1 -> PID Controller/1
  pqr_ref/1 -> Subsystem/1(pqr_ref)
  Demux/3 -> LowPass Filter1/1(raw_val)
  LowPass Filter1/1(filtered_val) -> Mux/3
  Demux/1 -> Mux/1
  Demux/2 -> Mux/2

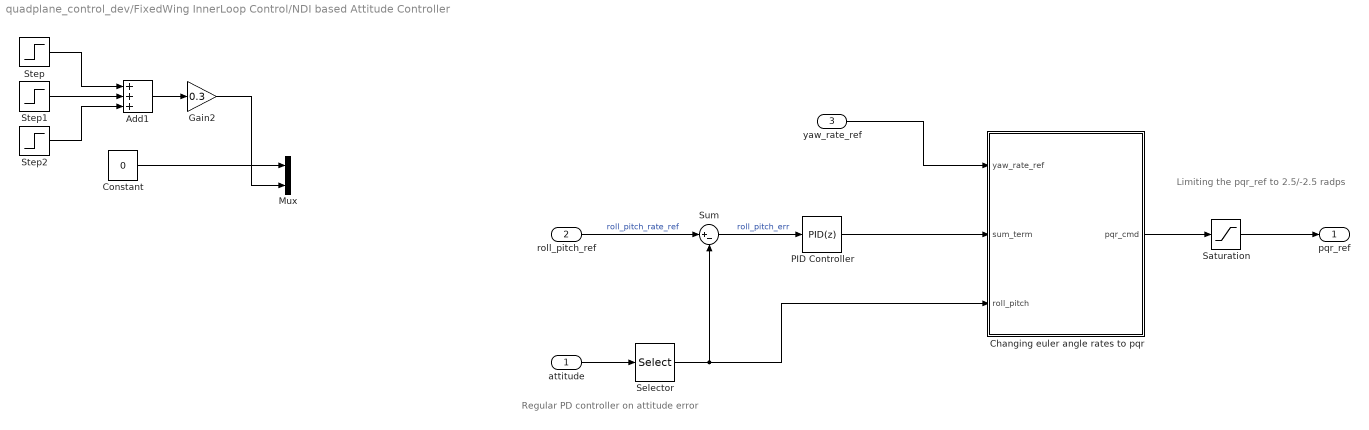
== system quadplane_control_dev/FixedWing InnerLoop Control/NDI based Attitude Controller ==
  note: Regular PD controller on attitude error
  note: Limiting the pqr_ref to 2.5/-2.5 radps
  attitude : Inport
  roll_pitch_ref : Inport  Port=2
  yaw_rate_ref : Inport  Port=3
  Add1 : Sum  Inputs=+++
  Changing euler angle rates to pqr : MATLAB Function  TreatAsAtomicUnit=on
  Constant : Constant  Value=0  OutDataTypeStr=single
  Gain2 : Gain  Gain=0.3
  Mux : Mux  Inputs=2
  PID Controller : slpidlib/PID Controller  Controller=PID  Form=Parallel  TimeDomain=Discrete-time  UseExternalTs=off  SampleTime=-1  IntegratorMethod=Forward Euler  FilterMethod=Forward Euler  ControllerParametersSource=internal  P=[3, 3.75]  I=[2.5, 0]  UseKiTs=off  D=[0, 0.1]  N=100  UseFilter=on  TunerSelectOption=Transfer Function Based (PID Tuner App)  InitialConditionSource=internal  InitialConditionForIntegrator=0  InitialConditionForFilter=0  DifferentiatorICPrevScaledInput=0  ExternalReset=none  TrackingMode=off  Kt=1  LimitOutput=off  SatLimitsSource=internal  UpperSaturationLimit=inf  LowerSaturationLimit=-inf  LinearizeAsGain=on  AntiWindupMode=none  Kb=1  LimitIntegrator=off  UpperIntegratorSaturationLimit=inf  LowerIntegratorSaturationLimit=-inf  POutMin=[]  POutMax=[]  IOutMin=[]  IOutMax=[]  DOutMin=[]  DOutMax=[]  NOutMin=[]  NOutMax=[]  SumOutMin=[]  SumOutMax=[]  SaturationOutMin=[]  SaturationOutMax=[]  PParamMin=[]  PParamMax=[]  IParamMin=[]  IParamMax=[]  DParamMin=[]  DParamMax=[]  NParamMin=[]  NParamMax=[]  KbParamMin=[]  KbParamMax=[]  KtParamMin=[]  KtParamMax=[]  KbOutMin=[]  KbOutMax=[]  KtOutMin=[]  KtOutMax=[]  IntegratorOutMin=[]  IntegratorOutMax=[]  FilterOutMin=[]  FilterOutMax=[]  SumI1OutMin=[]  SumI1OutMax=[]  SumI2OutMin=[]  SumI2OutMax=[]  SumI3OutMin=[]  SumI3OutMax=[]  SumI4OutMin=[]  SumI4OutMax=[]  SumDOutMin=[]  SumDOutMax=[]  DifferentiatorOutMin=[]  DifferentiatorOutMax=[]  FilterDiffOutCoefMin=[]  FilterDiffOutCoefMax=[]  ReciprocalOutMin=[]  ReciprocalOutMax=[]  SumDenOutMin=[]  SumDenOutMax=[]  SumNumOutMin=[]  SumNumOutMax=[]  DivideOutMin=[]  DivideOutMax=[]  UdiffTsProdOutMin=[]  UdiffTsProdOutMax=[]  NTsProdOutMin=[]  NTsProdOutMax=[]  UintegralTsProdOutMin=[]  UintegralTsProdOutMax=[]  UngainTsProdOutMin=[]  UngainTsProdOutMax=[]  ClampingZeroOutDataTypeStr=Inherit: Inherit via back propagation  ClampingZeroOutMin=[]  ClampingZeroOutMax=[]  FilterDenConstantOutDataTypeStr=Inherit: Inherit via back propagation  FilterDenConstantOutMin=[]  FilterDenConstantOutMax=[]  PCopyOutDataTypeStr=Inherit: Inherit via back propagation  PCopyOutMin=[]  PCopyOutMax=[]  NCopyOutDataTypeStr=Inherit: Inherit via back propagation  NCopyOutMin=[]  NCopyOutMax=[]  IntegratorContinuousStateAttributes=''  IntegratorStateMustResolveToSignalObject=off  IntegratorRTWStateStorageClass=Auto  FilterContinuousStateAttributes=''  FilterStateMustResolveToSignalObject=off  FilterRTWStateStorageClass=Auto  ParallelPVariant=InternalParameters  IdealPVariant=Disabled  IVariant=InternalParameters  DVariant=InternalParameters  IntegratorVariant=Discrete  SatVariant=Disabled  AWVariant=Passthrough  PCopyVariant=Disabled  TRVariant=Disabled  FdbkBlocksVariant=Forward  IdealPFdbkVariant=Disabled  SatFdbkVariant=Disabled  DerivativeFilterVariant=ForwardEulerFilter  NVariant=InternalParameters  NCopyVariant=Disabled  FilterICVariant=InternalICsFilter  IntegratorICVariant=InternalICs  ExternalResetVariant=Disabled  TRSumVariant=Passthrough  SumFdbkVariant=Disabled  SumVariant=Sum_PID  TsampFilterVariant=InternalTs  TsampNgainVariant=Passthrough  TsampIntegralVariant=Disabled_SignalSpec  ExternalSaturationOutDataTypeStr=Inherit: Same as second input
  Saturation : Saturate  UpperLimit=Aircraft.Control.Forward.max_pqr_ref  LowerLimit=-Aircraft.Control.Forward.max_pqr_ref
  Selector : Selector  InputPortWidth=3  IndexOptions=Index vector (dialog)  Indices=[1 2]  OutputSizes=1
  Step : Step  Time=3  OutDataTypeStr=single  SampleTime=0
  Step1 : Step  Time=7  Before=1  After=-1  OutDataTypeStr=single  SampleTime=0
  Step2 : Step  Time=11  Before=-1  After=0  OutDataTypeStr=single  SampleTime=0
  Sum : Sum  Inputs=|+-  AccumDataTypeStr=single
  pqr_ref : Outport
  wires:
  Changing euler angle rates to pqr/1(pqr_cmd) -> Saturation/1
  Saturation/1 -> pqr_ref/1
  yaw_rate_ref/1 -> Changing euler angle rates to pqr/1(yaw_rate_ref)
  Sum/1 -> PID Controller/1  "roll_pitch_err"
  PID Controller/1 -> Changing euler angle rates to pqr/2(sum_term)
  attitude/1 -> Selector/1
  Selector/1 -> Sum/2, Changing euler angle rates to pqr/3(roll_pitch)
  Add1/1 -> Gain2/1
  Step2/1 -> Add1/3
  Step1/1 -> Add1/2
  Step/1 -> Add1/1
  Gain2/1 -> Mux/2
  Constant/1 -> Mux/1
  roll_pitch_ref/1 -> Sum/1  "roll_pitch_rate_ref"

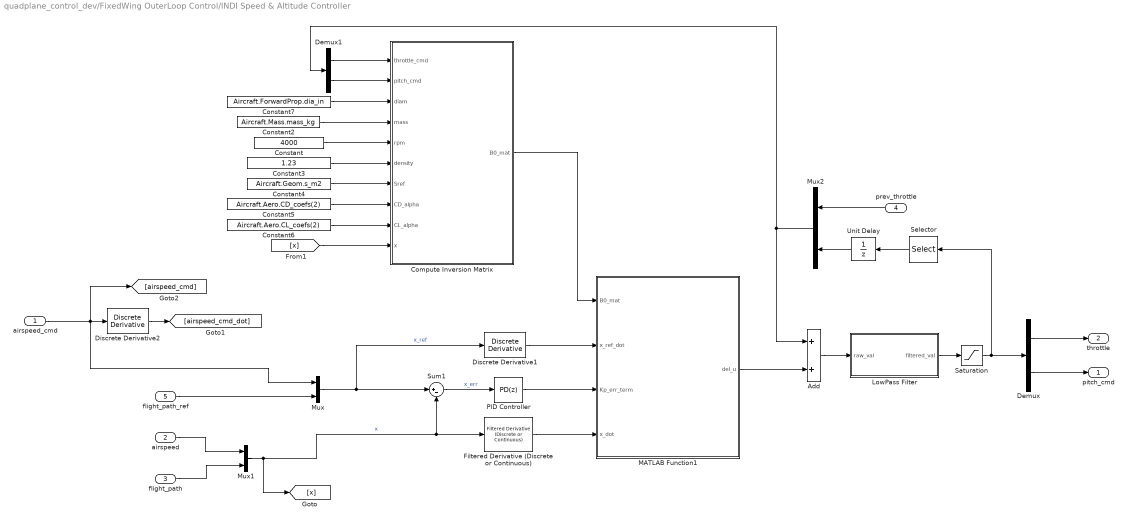
== system quadplane_control_dev/FixedWing OuterLoop Control/INDI Speed & Altitude Controller ==
  airspeed_cmd : Inport
  airspeed : Inport  Port=2
  flight_path : Inport  Port=3
  prev_throttle : Inport  Port=4
  flight_path_ref : Inport  Port=5
  Add : Sum  OutDataTypeStr=single
  Compute Inversion Matrix : MATLAB Function  TreatAsAtomicUnit=on
  Constant : Constant  Value=4000  OutDataTypeStr=single
  Constant2 : Constant  Value=Aircraft.Mass.mass_kg  OutDataTypeStr=single
  Constant3 : Constant  Value=1.23  OutDataTypeStr=single
  Constant4 : Constant  Value=Aircraft.Geom.s_m2  OutDataTypeStr=single
  Constant5 : Constant  Value=Aircraft.Aero.CD_coefs(2)  OutDataTypeStr=single
  Constant6 : Constant  Value=Aircraft.Aero.CL_coefs(2)  OutDataTypeStr=single
  Constant7 : Constant  Value=Aircraft.ForwardProp.dia_in  OutDataTypeStr=single
  Demux : Demux  Outputs=2
  Demux1 : Demux  Outputs=2
  Discrete Derivative1 : simulink/Discrete/Discrete Derivative  gainval=1.0  ICPrevScaledInput=0.0  OutMin=[]  OutMax=[]  OutDataType=fixdt(1, 16)  OutScaling=2^-10  DoSatur=off
  Discrete Derivative2 : simulink/Discrete/Discrete Derivative  gainval=1.0  ICPrevScaledInput=0.0  OutMin=[]  OutMax=[]  OutDataType=fixdt(1, 16)  OutScaling=2^-10  DoSatur=off
  Filtered Derivative (Discrete or Continuous) : eeGeneralControl/Filtered Derivative (Discrete or Continuous)  K=1  T=0.1  B=inf  A=-inf  minRatio=10  init_option=Inherited from block input  x0=0  Ts=-1
      settings: LibrarySourceBlock=|
      | ee_sl_lib/General Control/Filtered Derivative
      | (Discrete or Continuous)
  LowPass Filter : Subsystem
  MATLAB Function1 : MATLAB Function  TreatAsAtomicUnit=on
  Mux : Mux  Inputs=2
  Mux1 : Mux  Inputs=2
  Mux2 : Mux  Inputs=2
  PID Controller : slpidlib/PID Controller  Controller=PD  Form=Parallel  TimeDomain=Discrete-time  UseExternalTs=off  SampleTime=-1  IntegratorMethod=Forward Euler  FilterMethod=Forward Euler  ControllerParametersSource=internal  P=[1.2, 3]  I=1  UseKiTs=off  D=[0, 2]  N=5  UseFilter=off  TunerSelectOption=Transfer Function Based (PID Tuner App)  InitialConditionSource=internal  InitialConditionForIntegrator=0  InitialConditionForFilter=0  DifferentiatorICPrevScaledInput=0  ExternalReset=none  TrackingMode=off  Kt=1  LimitOutput=off  SatLimitsSource=internal  UpperSaturationLimit=inf  LowerSaturationLimit=-inf  LinearizeAsGain=on  AntiWindupMode=none  Kb=1  LimitIntegrator=off  UpperIntegratorSaturationLimit=inf  LowerIntegratorSaturationLimit=-inf  POutMin=[]  POutMax=[]  IOutMin=[]  IOutMax=[]  DOutMin=[]  DOutMax=[]  NOutMin=[]  NOutMax=[]  SumOutMin=[]  SumOutMax=[]  SaturationOutMin=[]  SaturationOutMax=[]  PParamMin=[]  PParamMax=[]  IParamMin=[]  IParamMax=[]  DParamMin=[]  DParamMax=[]  NParamMin=[]  NParamMax=[]  KbParamMin=[]  KbParamMax=[]  KtParamMin=[]  KtParamMax=[]  KbOutMin=[]  KbOutMax=[]  KtOutMin=[]  KtOutMax=[]  IntegratorOutMin=[]  IntegratorOutMax=[]  FilterOutMin=[]  FilterOutMax=[]  SumI1OutMin=[]  SumI1OutMax=[]  SumI2OutMin=[]  SumI2OutMax=[]  SumI3OutMin=[]  SumI3OutMax=[]  SumI4OutMin=[]  SumI4OutMax=[]  SumDOutMin=[]  SumDOutMax=[]  DifferentiatorOutMin=[]  DifferentiatorOutMax=[]  FilterDiffOutCoefMin=[]  FilterDiffOutCoefMax=[]  ReciprocalOutMin=[]  ReciprocalOutMax=[]  SumDenOutMin=[]  SumDenOutMax=[]  SumNumOutMin=[]  SumNumOutMax=[]  DivideOutMin=[]  DivideOutMax=[]  UdiffTsProdOutMin=[]  UdiffTsProdOutMax=[]  NTsProdOutMin=[]  NTsProdOutMax=[]  UintegralTsProdOutMin=[]  UintegralTsProdOutMax=[]  UngainTsProdOutMin=[]  UngainTsProdOutMax=[]  ClampingZeroOutDataTypeStr=Inherit: Inherit via back propagation  ClampingZeroOutMin=[]  ClampingZeroOutMax=[]  FilterDenConstantOutDataTypeStr=Inherit: Inherit via back propagation  FilterDenConstantOutMin=[]  FilterDenConstantOutMax=[]  PCopyOutDataTypeStr=Inherit: Inherit via back propagation  PCopyOutMin=[]  PCopyOutMax=[]  NCopyOutDataTypeStr=Inherit: Inherit via back propagation  NCopyOutMin=[]  NCopyOutMax=[]  IntegratorContinuousStateAttributes=''  IntegratorStateMustResolveToSignalObject=off  IntegratorRTWStateStorageClass=Auto  FilterContinuousStateAttributes=''  FilterStateMustResolveToSignalObject=off  FilterRTWStateStorageClass=Auto  ParallelPVariant=InternalParameters  IdealPVariant=Disabled  IVariant=Disabled  DVariant=InternalParameters  IntegratorVariant=Disabled  SatVariant=Disabled  AWVariant=Disabled  PCopyVariant=Disabled  TRVariant=Disabled  FdbkBlocksVariant=Forward  IdealPFdbkVariant=Disabled  SatFdbkVariant=Disabled  DerivativeFilterVariant=Differentiator  NVariant=Passthrough  NCopyVariant=Disabled_SignalSpec  FilterICVariant=InternalICsDifferentiator  IntegratorICVariant=Disabled  ExternalResetVariant=Disabled  TRSumVariant=Passthrough  SumFdbkVariant=Disabled  SumVariant=Sum_PD  TsampFilterVariant=InternalTs  TsampNgainVariant=Passthrough  TsampIntegralVariant=Disabled_SignalSpec  ExternalSaturationOutDataTypeStr=Inherit: Same as second input
  Saturation : Saturate  UpperLimit=[1, Aircraft.Control.Forward.max_pitch_rad]'  LowerLimit=[0, -Aircraft.Control.Forward.max_pitch_rad]'
  Selector : Selector  InputPortWidth=2  IndexOptions=Index vector (dialog)  Indices=2  OutputSizes=1
  Sum1 : Sum  Inputs=|+-
  Unit Delay : UnitDelay  SampleTime=-1  HasFrameUpgradeWarning=on
  pitch_cmd : Outport
  throttle : Outport  Port=2
  wires:
  Constant5/1 -> Compute Inversion Matrix/8(CD_alpha)
  Demux/2 -> pitch_cmd/1
  Constant/1 -> Compute Inversion Matrix/5(rpm)
  prev_throttle/1 -> Mux2/1
  Mux2/1 -> Demux1/1, Add/1
  Discrete Derivative1/1 -> MATLAB Function1/2(x_ref_dot)
  Unit Delay/1 -> Mux2/2
  Compute Inversion Matrix/1(B0_mat) -> MATLAB Function1/1(B0_mat)
  Filtered Derivative (Discrete or Continuous)/1 -> MATLAB Function1/4(x_dot)
  Constant2/1 -> Compute Inversion Matrix/4(mass)
  Saturation/1 -> Selector/1, Demux/1
  Selector/1 -> Unit Delay/1
  Constant7/1 -> Compute Inversion Matrix/3(diam)
  Add/1 -> LowPass Filter/1(raw_val)
  Demux1/1 -> Compute Inversion Matrix/1(throttle_cmd)
  Demux1/2 -> Compute Inversion Matrix/2(pitch_cmd)
  Mux1/1 -> Filtered Derivative (Discrete or Continuous)/1, Sum1/2, [x]  "x"
  LowPass Filter/1(filtered_val) -> Saturation/1
  Constant6/1 -> Compute Inversion Matrix/9(CL_alpha)
  [x] -> Compute Inversion Matrix/10(x)
  Constant4/1 -> Compute Inversion Matrix/7(Sref)
  Constant3/1 -> Compute Inversion Matrix/6(density)
  MATLAB Function1/1(del_u) -> Add/2
  Sum1/1 -> PID Controller/1  "x_err"
  PID Controller/1 -> MATLAB Function1/3(Kp_err_term)
  Mux/1 -> Sum1/1, Discrete Derivative1/1  "x_ref"
  airspeed_cmd/1 -> Discrete Derivative2/1, [airspeed_cmd], Mux/1
  Discrete Derivative2/1 -> [airspeed_cmd_dot]
  Demux/1 -> throttle/1
  airspeed/1 -> Mux1/1
  flight_path/1 -> Mux1/2
  flight_path_ref/1 -> Mux/2
